simulink model "SensorFaultInj"  (R2014a)
settings: Solver=FixedStepDiscrete  SolverMode=SingleTasking  StartTime=0.0  StopTime=SimLength  FixedStep=SampleTime  RelTol=1e-3
values from neighbouring files (symbols this model uses):
  GlobalSeed = 10    [set_global_attr.m]
  SampleTime = 0.01    [set_global_attr.m]
  SimLength = 40    [set_global_attr.m]
undefined symbols (not defined in the file or in its folder): actMat, DiscIntNeverNeededParam
libraries: simulink x16, dspswit3 x10
(part 1 of 4)
settings Model: Creator=Maik  LastModifiedBy=Maik
settings DataIOCC: SaveOutput=off  SaveTime=off
settings DebuggingCC: UnconnectedOutputMsg=none  BusObjectLabelMismatch=none  StateNameClashWarn=warning

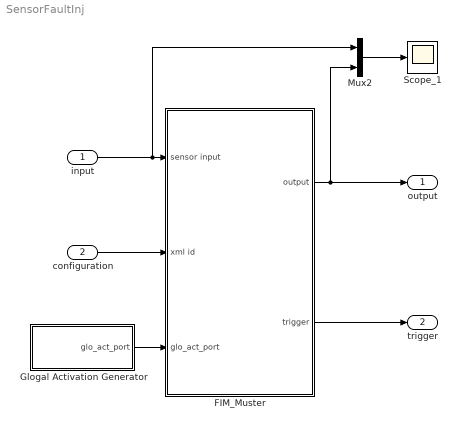
== system SensorFaultInj ==
  "input " : Inport  SampleTime=SampleTime
  configuration : Inport  Port=2  OutDataTypeStr=single  SampleTime=SampleTime
  FIM_Muster : Subsystem
  Glogal Activation Generator : Subsystem  TreatAsAtomicUnit=on
  Mux2 : Mux  Inputs=2
  Scope_1 : Scope
      settings: TimeRange=40  YMin=0.1  YMax=0.24  SaveName=SensordataEva01  MaxDataPoints=50000
  output : Outport
  trigger : Outport  Port=2  OutDataTypeStr=Bus: TriggerBus  SampleTime=SampleTime
  wires:
  Mux2/1 -> Scope_1/1
  FIM_Muster/1(output) -> Mux2/2, output/1
  "input "/1 -> Mux2/1, FIM_Muster/1(sensor input)
  configuration/1 -> FIM_Muster/2(xml id)
  Glogal Activation Generator/1(glo_act_port) -> FIM_Muster/3(glo_act_port)
  FIM_Muster/2(trigger) -> trigger/1

== system SensorFaultInj/FIM_Muster ==
  sensor input : Inport
  xml id : Inport  Port=2  SampleTime=SampleTime
  glo_act_port : Inport  Port=3
  Fault Injection Modul : Subsystem
  Local Activation Generator : Subsystem
  Parser Modul : Subsystem
  logger : Subsystem
  trigger signal generation : Subsystem
  output : Outport
  trigger : Outport  Port=2
  wires:
  Parser Modul/1(schedule_port) -> Local Activation Generator/1(schedule_port), trigger signal generation/1(schedule), Fault Injection Modul/2(schedule_port)
  Parser Modul/2(occurrnce_port) -> Local Activation Generator/2(occurrence_port)
  Local Activation Generator/1(activation_port) -> Parser Modul/2("actiavtion_vector "), trigger signal generation/2(activation), Fault Injection Modul/3(activation_port)
  Fault Injection Modul/1(Out1) -> logger/2("input "), output/1
  sensor input/1 -> Fault Injection Modul/1(sensor input)
  xml id/1 -> logger/1(xml_id), Parser Modul/1(xml id)
  Parser Modul/3(parameter_port) -> Local Activation Generator/3("param_port "), Fault Injection Modul/4(parameter_port)
  Fault Injection Modul/2("amplitude_port ") -> logger/4("amp_port ")
  Local Activation Generator/2(log_port) -> logger/3("act_port ")
  glo_act_port/1 -> Local Activation Generator/4(glo_act_port)
  trigger signal generation/1(Out1) -> trigger/1

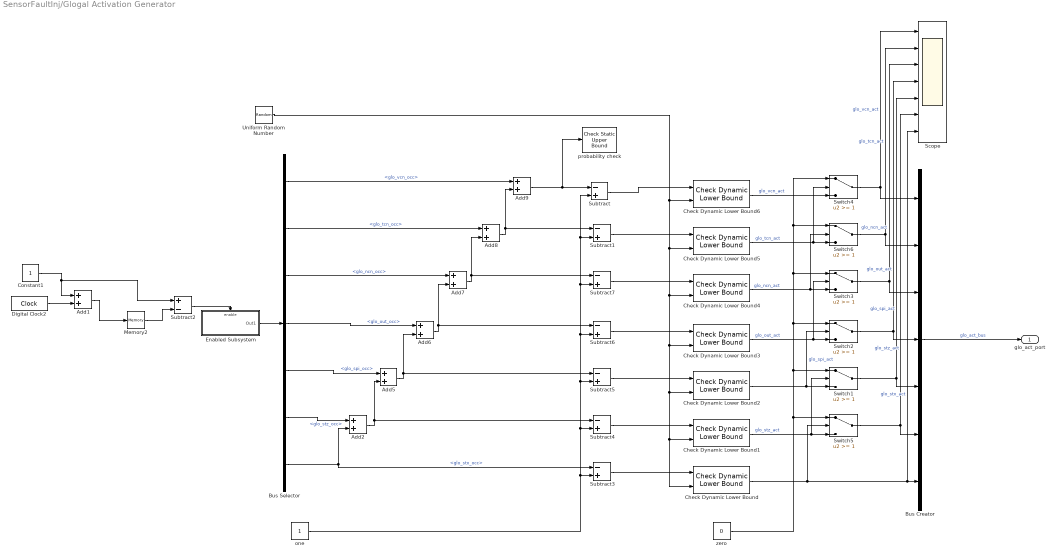
== system SensorFaultInj/Glogal Activation Generator ==
  Add{1..2,5..9} (7 alike) : Sum
  Bus Creator : BusCreator  Inputs=7
  Bus Selector : BusSelector  OutputSignals=glo_vcn_occ,glo_tcn_occ,glo_ncn_occ,glo_out_occ,glo_spi_occ,glo_stz_occ,glo_stx_occ
  Check Dynamic Lower Bound{,1..6} (7 alike) : simulink/Model Verification/Check Dynamic  Lower Bound  Description=min < sig  Enabled=off  stopWhenAssertionFail=off  export=on  icon=graphic
  Constant1 : Constant
  Digital Clock2 : DigitalClock  SampleTime=SampleTime
  Enabled Subsystem : Subsystem  TreatAsAtomicUnit=on
  Memory2 : Memory
  Scope : Scope  NumInputPorts=7
      settings: YMin=-5~-5~-5~-5~-5~-5~-5  YMax=5~5~5~5~5~5~5  SaveName=ScopeData10
  Subtract{,1,3..7} (7 alike) : Sum  Inputs=-+
  Subtract2 : Sum  Inputs=+-
  Switch{1..6} (6 alike) : Switch  Threshold=1
      settings: LockScale=on
  Uniform Random Number : UniformRandomNumber  Seed=GlobalSeed  SampleTime=SampleTime
  one : Constant
  probability check : simulink/Model Verification/Check Static  Upper Bound  Description=u <= 1  max=1  max_included=on  enabled=on  stopWhenAssertionFail=on  export=off  icon=graphic
  zero : Constant  Value=0
  glo_act_port : Outport
  wires:
  Bus Selector/7 -> Subtract3/1, Add2/2  "<glo_stx_occ>"
  Bus Selector/6 -> Add2/1  "<glo_stz_occ>"
  Add5/1 -> Add6/2, Subtract5/1
  Bus Selector/5 -> Add5/1  "<glo_spi_occ>"
  Bus Selector/4 -> Add6/1  "<glo_out_occ>"
  Add6/1 -> Add7/2, Subtract6/1
  Add7/1 -> Add8/2, Subtract7/1
  Bus Selector/3 -> Add7/1  "<glo_ncn_occ>"
  Bus Selector/2 -> Add8/1  "<glo_tcn_occ>"
  Add8/1 -> Add9/2, Subtract1/1
  Bus Selector/1 -> Add9/1  "<glo_vcn_occ>"
  Uniform Random Number/1 -> Check Dynamic Lower Bound/2, Check Dynamic Lower Bound1/2, Check Dynamic Lower Bound2/2, Check Dynamic Lower Bound3/2, Check Dynamic Lower Bound4/2, Check Dynamic Lower Bound5/2, Check Dynamic Lower Bound6/2
  Subtract/1 -> Check Dynamic Lower Bound6/1
  Add9/1 -> probability check/1, Subtract/1
  Subtract1/1 -> Check Dynamic Lower Bound5/1
  Subtract7/1 -> Check Dynamic Lower Bound4/1
  Subtract6/1 -> Check Dynamic Lower Bound3/1
  Subtract5/1 -> Check Dynamic Lower Bound2/1
  Subtract4/1 -> Check Dynamic Lower Bound1/1
  Subtract3/1 -> Check Dynamic Lower Bound/1
  one/1 -> Subtract/2, Subtract1/2, Subtract7/2, Subtract6/2, Subtract5/2, Subtract4/2, Subtract3/2
  Add2/1 -> Subtract4/1, Add5/2
  Check Dynamic Lower Bound/1 -> Switch5/2, Scope/7, Bus Creator/7  "glo_stx_act"
  Switch5/1 -> Bus Creator/6, Scope/6  "glo_stz_act"
  Switch1/1 -> Bus Creator/5, Scope/5  "glo_spi_act"
  Switch2/1 -> Bus Creator/4, Scope/4  "glo_out_act"
  Switch3/1 -> Bus Creator/3, Scope/3  "glo_ncn_act"
  Switch6/1 -> Bus Creator/2, Scope/2  "glo_tcn_act"
  Switch4/1 -> Bus Creator/1, Scope/1  "glo_vcn_act"
  Bus Creator/1 -> glo_act_port/1  "glo_act_bus"
  Check Dynamic Lower Bound1/1 -> Switch1/2, Switch5/3  "glo_stz_act"
  zero/1 -> Switch3/1, Switch6/1, Switch4/1, Switch2/1, Switch1/1, Switch5/1
  Check Dynamic Lower Bound2/1 -> Switch2/2, Switch1/3  "glo_spi_act"
  Check Dynamic Lower Bound3/1 -> Switch3/2, Switch2/3  "glo_out_act"
  Check Dynamic Lower Bound4/1 -> Switch6/2, Switch3/3  "glo_ncn_act"
  Check Dynamic Lower Bound5/1 -> Switch4/2, Switch6/3  "glo_tcn_act"
  Check Dynamic Lower Bound6/1 -> Switch4/3  "glo_vcn_act"
  Digital Clock2/1 -> Add1/2
  Memory2/1 -> Subtract2/2
  Constant1/1 -> Add1/1, Subtract2/1
  Add1/1 -> Memory2/1
  Subtract2/1 -> Enabled Subsystem/Enable
  Enabled Subsystem/1(Out1) -> Bus Selector/1

== system SensorFaultInj/FIM_Muster/Fault Injection Modul ==
  sensor input : Inport
  schedule_port : Inport  Port=2
  activation_port : Inport  Port=3
  parameter_port : Inport  Port=4
  AFI - additive faults injection : Subsystem
  Bus Creator : BusCreator  Inputs=3
  FFI - functional fault injection : Subsystem
  MFI - multiplicative fault injection : Subsystem
  activation bus creator : Subsystem
  schedule bus creator : Subsystem
  schedule bus creator1 : Subsystem
  Out1 : Outport
  "amplitude_port " : Outport  Port=2
  wires:
  MFI - multiplicative fault injection/1(output) -> AFI - additive faults injection/1(input)
  FFI - functional fault injection/1(output) -> Out1/1
  AFI - additive faults injection/1(output) -> FFI - functional fault injection/1(input)
  sensor input/1 -> MFI - multiplicative fault injection/1(In1)
  activation_port/1 -> activation bus creator/1(act_port)
  schedule_port/1 -> schedule bus creator/1(schedule_port)
  schedule bus creator/1(mfi_sched_port) -> MFI - multiplicative fault injection/2(sched_port)
  activation bus creator/1(mfi_act_port) -> MFI - multiplicative fault injection/3(act_port)
  schedule bus creator1/1(mfi_sched_port) -> MFI - multiplicative fault injection/4(param_port)
  schedule bus creator/2(afi_sched_port) -> AFI - additive faults injection/2(sched_bus)
  activation bus creator/2(afi_act_port) -> AFI - additive faults injection/3(act_bus)
  schedule bus creator1/2(afi_sched_port) -> AFI - additive faults injection/4(param_bus)
  schedule bus creator/3(ffi_sched_port) -> FFI - functional fault injection/2(schedule_port)
  schedule bus creator1/3(ffi_sched_port) -> FFI - functional fault injection/3(param_port)
  parameter_port/1 -> schedule bus creator1/1(schedule_port)
  MFI - multiplicative fault injection/2("amplitude_port ") -> Bus Creator/1
  AFI - additive faults injection/2("amplitude_bus ") -> Bus Creator/2
  Bus Creator/1 -> "amplitude_port "/1  "ampl_bus"
  FFI - functional fault injection/2(amplitude_port) -> Bus Creator/3

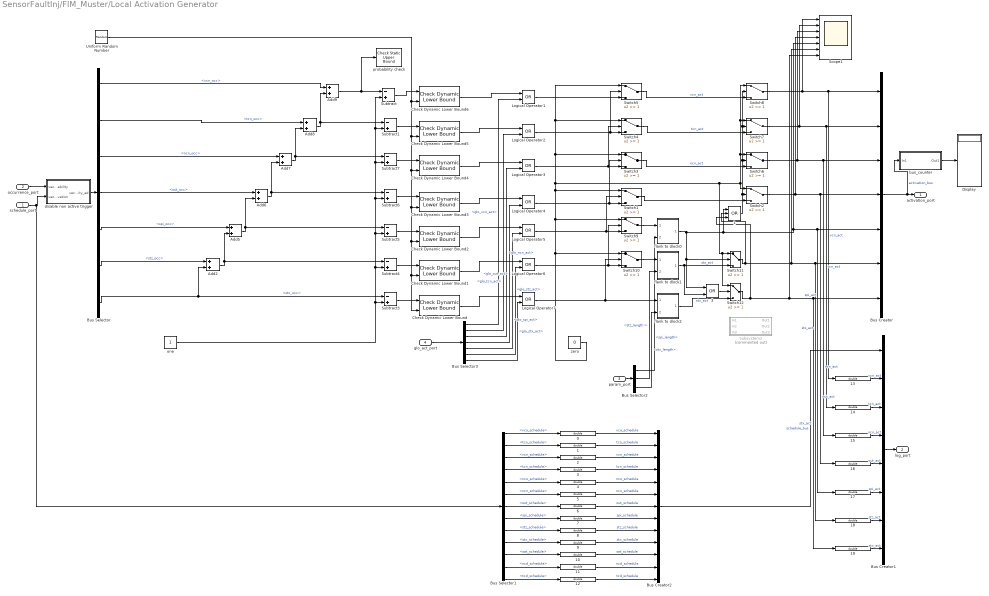
== system SensorFaultInj/FIM_Muster/Local Activation Generator ==
  schedule_port : Inport
  occurrence_port : Inport  Port=2
  "param_port " : Inport  Port=3
  glo_act_port : Inport  Port=4
  " 1" : Logic  Operator=OR  Inputs=3  AllPortsSameDT=off  OutDataTypeStr=boolean
  " 3" : Logic  Operator=OR  AllPortsSameDT=off  OutDataTypeStr=boolean
  {0..19} (20 alike) : DataTypeConversion  OutDataTypeStr=double
  Add{2,5..9} (6 alike) : Sum
  Bus Creator : BusCreator  Inputs=7
  Bus Creator1 : BusCreator  Inputs=8
  Bus Creator2 : BusCreator  Inputs=13
  Bus Selector : BusSelector  OutputSignals=vcn_occ,tcn_occ,ncn_occ,out_occ,spi_occ,stz_occ,stx_occ
  Bus Selector1 : BusSelector  OutputSignals=vco_schedule,tco_schedule,vcn_schedule,tcn_schedule,nco_schedule,ncn_schedule,out_schedule,spi_schedule,stz_schedule,stx_schedule,sat_schedule,ncd_schedule,tcd_schedule
  Bus Selector2 : BusSelector  OutputSignals=parameter_bus.spi_param_bus.spi_length,parameter_bus.stz_length ,parameter_bus.stx_param_bus.stx_length
  Bus Selector3 : BusSelector  OutputSignals=glo_vcn_act,glo_tcn_act,glo_ncn_act,glo_out_act,glo_spi_act,glo_stz_act,glo_stx_act
  Check Dynamic Lower Bound{,1..6} (7 alike) : simulink/Model Verification/Check Dynamic  Lower Bound  Description=min < sig  Enabled=off  stopWhenAssertionFail=off  export=on  icon=graphic
  Display : Display
  Logical Operator{1..7} (7 alike) : Logic  Operator=OR  AllPortsSameDT=off  OutDataTypeStr=boolean
  Scope1 : Scope  NumInputPorts=7
      settings: TimeRange=1  YMin=-1~0~-5~-5~-5~-5~-5  YMax=1~1~5~5~5~5~5  SaveName=ScopeData23  MaxDataPoints=50000
  Subsystem2 : Subsystem  Commented=on
  Subtract{,1,3..7} (7 alike) : Sum  Inputs=-+
  Switch{1..12} (12 alike) : Switch  Threshold=1
      Switch1 settings: LockScale=on
      Switch10 settings: LockScale=on
      Switch5 settings: LockScale=on
      Switch9 settings: LockScale=on
  Uniform Random Number : UniformRandomNumber  Minimum=0  Seed=1  SampleTime=SampleTime
  bus_counter : Subsystem
  disable non active trigger : Subsystem
  flank to dlock0 : Subsystem
  flank to dlock1 : Subsystem
  flank to dlock2 : Subsystem
  one : Constant
  probability check : simulink/Model Verification/Check Static  Upper Bound  Description=u <= 1  max=1  max_included=on  enabled=on  stopWhenAssertionFail=on  export=off  icon=graphic
  zero : Constant  Value=0  OutDataTypeStr=boolean
  activation_port : Outport
  log_port : Outport  Port=2
  wires:
  Bus Selector/7 -> Add2/2, Subtract3/1  "<stx_occ>"
  Bus Selector/6 -> Add2/1  "<stz_occ>"
  Add5/1 -> Add6/2, Subtract5/1
  Bus Selector/5 -> Add5/1  "<spi_occ>"
  Bus Selector/4 -> Add6/1  "<out_occ>"
  Add6/1 -> Add7/2, Subtract6/1
  Add7/1 -> Add8/2, Subtract7/1
  Bus Selector/3 -> Add7/1  "<ncn_occ>"
  Bus Selector/2 -> Add8/1  "<tcn_occ>"
  Add8/1 -> Add9/2, Subtract1/1
  Bus Selector/1 -> Add9/1  "<vcn_occ>"
  Subtract/1 -> Check Dynamic Lower Bound6/1
  Add9/1 -> probability check/1, Subtract/1
  Subtract1/1 -> Check Dynamic Lower Bound5/1
  Subtract7/1 -> Check Dynamic Lower Bound4/1
  Subtract6/1 -> Check Dynamic Lower Bound3/1
  Subtract5/1 -> Check Dynamic Lower Bound2/1
  Subtract4/1 -> Check Dynamic Lower Bound1/1
  Subtract3/1 -> Check Dynamic Lower Bound/1
  one/1 -> Subtract/2, Subtract1/2, Subtract7/2, Subtract6/2, Subtract5/2, Subtract4/2, Subtract3/2
  zero/1 -> Switch1/1, Switch12/1, Switch11/1, Switch2/1, Switch8/1, Switch7/1, Switch6/1, Switch3/1, Switch4/1, Switch5/1, Switch9/1, Switch10/1
  Switch8/1 -> Scope1/1, 13/1, Bus Creator/1  "vcn_act"
  Switch7/1 -> Scope1/2, 14/1, Bus Creator/2  "tcn_act"
  Switch6/1 -> Scope1/3, 15/1, Bus Creator/3  "ncn_act"
  Switch2/1 -> 16/1, Bus Creator/4, Scope1/4  "out_act"
  flank to dlock0/1(block) -> " 1"/1, Scope1/5, 17/1, Bus Creator/5, Switch11/2, " 3"/1  "spi_act"
  Switch11/1 -> " 1"/2, Scope1/6, 18/1, Bus Creator/6  "stz_act"
  Bus Creator/1 -> activation_port/1, bus_counter/1(In1)  "activation_bus"
  occurrence_port/1 -> disable non active trigger/1(vec_probability)
  schedule_port/1 -> Bus Selector1/1, disable non active trigger/2(vec_activation)
  Add2/1 -> Subtract4/1, Add5/2
  Switch12/1 -> " 1"/3, Scope1/7, 19/1, Bus Creator/7  "stx_act"
  disable non active trigger/1(vec_probability_ad) -> Bus Selector/1
  Bus Creator1/1 -> log_port/1
  Bus Selector1/1 -> 0/1  "<vco_schedule>"
  3/1 -> Bus Creator2/4  "tcn_schedule"
  0/1 -> Bus Creator2/1  "vco_schedule"
  4/1 -> Bus Creator2/5  "nco_schedule"
  1/1 -> Bus Creator2/2  "tco_schedule"
  2/1 -> Bus Creator2/3  "vcn_schedule"
  5/1 -> Bus Creator2/6  "ncn_schedule"
  6/1 -> Bus Creator2/7  "out_schedule"
  12/1 -> Bus Creator2/13  "tcd_schedule"
  7/1 -> Bus Creator2/8  "spi_schedule"
  8/1 -> Bus Creator2/9  "stz_schedule"
  9/1 -> Bus Creator2/10  "stx_schedule"
  10/1 -> Bus Creator2/11  "sat_schedule"
  11/1 -> Bus Creator2/12  "ncd_schedule"
  Bus Selector1/2 -> 1/1  "<tco_schedule>"
  Bus Selector1/3 -> 2/1  "<vcn_schedule>"
  Bus Selector1/4 -> 3/1  "<tcn_schedule>"
  Bus Selector1/5 -> 4/1  "<nco_schedule>"
  Bus Selector1/6 -> 5/1  "<ncn_schedule>"
  Bus Selector1/7 -> 6/1  "<out_schedule>"
  Bus Selector1/8 -> 7/1  "<spi_schedule>"
  Bus Selector1/9 -> 8/1  "<stz_schedule>"
  Bus Selector1/10 -> 9/1  "<stx_schedule>"
  Bus Selector1/11 -> 10/1  "<sat_schedule>"
  Bus Selector1/12 -> 11/1  "<ncd_schedule>"
  Bus Selector1/13 -> 12/1  "<tcd_schedule>"
  Bus Creator2/1 -> Bus Creator1/1  "schedule_bus"
  13/1 -> Bus Creator1/2  "vcn_act"
  14/1 -> Bus Creator1/3  "tcn_act"
  15/1 -> Bus Creator1/4  "ncn_act"
  16/1 -> Bus Creator1/5  "out_act"
  17/1 -> Bus Creator1/6  "spi_act"
  18/1 -> Bus Creator1/7  "stz_act"
  19/1 -> Bus Creator1/8  "stx_act"
  "param_port "/1 -> Bus Selector2/1
  Bus Selector2/1 -> flank to dlock0/2(delay)  "<spi_length>"
  Bus Selector2/2 -> flank to dlock1/2(delay)  "<stz_length >"
  Bus Selector2/3 -> flank to dlock2/2(delay)  "<stx_length>"
  Logical Operator1/1 -> Switch5/3
  Check Dynamic Lower Bound6/1 -> Logical Operator1/1
  Logical Operator3/1 -> Switch3/3, Switch4/2
  Logical Operator2/1 -> Switch5/2, Switch4/3
  Check Dynamic Lower Bound5/1 -> Logical Operator2/1
  Check Dynamic Lower Bound4/1 -> Logical Operator3/1
  Check Dynamic Lower Bound3/1 -> Logical Operator4/1
  Check Dynamic Lower Bound2/1 -> Logical Operator5/1
  Check Dynamic Lower Bound1/1 -> Logical Operator6/1
  Check Dynamic Lower Bound/1 -> Logical Operator7/1
  glo_act_port/1 -> Bus Selector3/1
  Bus Selector3/7 -> Logical Operator7/2  "<glo_stx_act>"
  Bus Selector3/6 -> Logical Operator6/2  "<glo_stz_act>"
  Bus Selector3/5 -> Logical Operator5/2  "<glo_spi_act>"
  Bus Selector3/4 -> Logical Operator4/2  "<glo_out_act>"
  Bus Selector3/3 -> Logical Operator3/2  "<glo_ncn_act>"
  Bus Selector3/2 -> Logical Operator2/2  "<glo_tcn_act>"
  Bus Selector3/1 -> Logical Operator1/2  "<glo_vcn_act>"
  bus_counter/1(Out1) -> Display/1
  Uniform Random Number/1 -> Check Dynamic Lower Bound4/2, Check Dynamic Lower Bound3/2, Check Dynamic Lower Bound2/2, Check Dynamic Lower Bound1/2, Check Dynamic Lower Bound/2, Check Dynamic Lower Bound5/2, Check Dynamic Lower Bound6/2
  " 1"/1 -> Switch6/2, Switch8/2, Switch7/2, Switch2/2
  Switch3/1 -> Switch6/3  "ncn_act"
  Switch4/1 -> Switch7/3  "tcn_act"
  Switch5/1 -> Switch8/3  "vcn_act"
  Switch1/1 -> Switch2/3
  Logical Operator4/1 -> Switch3/2, Switch1/3
  Logical Operator5/1 -> Switch1/2, Switch9/3
  Logical Operator6/1 -> Switch9/2, Switch10/3
  Logical Operator7/1 -> flank to dlock2/1(flank), Switch10/2
  Switch10/1 -> flank to dlock1/1(flank)
  Switch9/1 -> flank to dlock0/1(flank)
  flank to dlock2/1(block) -> Switch12/3  "stx_act"
  flank to dlock1/1(block) -> " 3"/2, Switch11/3  "stz_act"
  " 3"/1 -> Switch12/2

== system SensorFaultInj/FIM_Muster/Parser Modul ==
  xml id : Inport
  "actiavtion_vector " : Inport  Port=2
  Bus Creator : BusCreator  Inputs=2
  Fault Parameter Parser : Subsystem
  "Occurence Parser " : Subsystem  Commented=on
  "Schedule Parser and Generator " : Subsystem
  "actication matrix parser " : Subsystem
  activation_vec : Display
  parameter_vec : Display
  schedule : Scope
      settings: SaveName=ScopeData2
  schedule_port : Outport
  occurrnce_port : Outport  Port=2
  parameter_port : Outport  Port=3
  wires:
  "Schedule Parser and Generator "/1(Out1) -> schedule/1, activation_vec/1, schedule_port/1
  xml id/1 -> "Schedule Parser and Generator "/1(In1), Fault Parameter Parser/1(In1), Bus Creator/2, "Occurence Parser "/1(In1)  "xml_id"
  Fault Parameter Parser/1(Out1) -> parameter_vec/1, Bus Creator/1  "parameter_bus"
  Bus Creator/1 -> parameter_port/1
  "actiavtion_vector "/1 -> "actication matrix parser "/1(In1)
  "actication matrix parser "/1(Out1) -> occurrnce_port/1

== system SensorFaultInj/FIM_Muster/logger ==
  xml_id : Inport
  "input " : Inport  Port=2
  "act_port " : Inport  Port=3
  "amp_port " : Inport  Port=4
  Bus Creator : BusCreator  Inputs=13
  Bus Creator1 : BusCreator  Inputs=13
  Bus Selector : BusSelector  OutputSignals=schedule_bus.vco_schedule,schedule_bus.tco_schedule,vcn_act,tcn_act,schedule_bus.nco_schedule,ncn_act,out_act,spi_act,stz_act,stx_act,schedule_bus.sat_schedule,schedule_bus.ncd_schedule,schedule_bus.tcd_schedule
  Bus Selector1 : BusSelector  OutputSignals=mfi_amp_bus.vco_ampl,mfi_amp_bus.tco_ampl,mfi_amp_bus.vcn_ampl,mfi_amp_bus.tcn_ampl,afi_ampl_bus.nco_ampl,afi_ampl_bus.ncn_ampl,afi_ampl_bus.out_ampl,afi_ampl_bus.spike_ampl,afi_ampl_bus.stz_ampl,afi_ampl_bus.stx_ampl,ffi_ampl_bus.sat_ampl,ffi_ampl_bus.ncd_ampl,ffi_ampl_bus.tcd_ampl
  Constant1 : Constant
  Discrete-Time Integrator : DiscreteIntegrator  SampleTime=SampleTime  ICPrevOutput=DiscIntNeverNeededParam  ICPrevScaledInput=DiscIntNeverNeededParam
  Display : Display
  Display1 : Display
  ex_sfun_logger : S-Function  FunctionName=ex_sfun_logger  EnableBusSupport=off  mask(Legacy Function){SFunctionSpec=single y1 = logger(single u1, double u2, double u3, double u4[], double u5[]), ShowSpec=on}
      mask prompts: ShowSpec "Display function specification"
      mask help:
      | This block allows you to call the legacy functions specified by the following Legacy Code Tool definition:
      | def.SFunctionName = 'ex_sfun_logger';
      | def.OutputFcnSpec = 'single y1 = logger(single u1, double u2, double u3, double u4[], double u5[])';
      | def.HeaderFiles = {'logger.hpp'};
      | def.SourceFiles = {'logger.cpp'};
      | def.Options.language = 'C++';
      mask Help: <p>This block was generated automatically by the Legacy Code Tool. For detailed help on this tool, call<a href="matlab:legacy_code('help')"> legacy_code('help')</a>.</p>
      mask Callback ShowSpec:
      | if strcmp(get_param(gcbh, 'ShowSpec'), 'on')
      |   set_param(gcbh, 'MaskDisplay', sprintf('fprintf(''%s'');', get_param(gcbh, 'SFunctionSpec')));
      | else
      |   set_param(gcbh, 'MaskDisplay', sprintf('fprintf(''%s'');', get_param(gcbh, 'FunctionName')));
      | end
      mask Display: fprintf('single y1 = logger(single u1, double u2, double u3, double u4[], double u5[])');
  wires:
  "act_port "/1 -> Bus Selector/1
  "amp_port "/1 -> Bus Selector1/1
  Bus Selector1/2 -> Bus Creator1/2  "<tco_ampl>"
  Bus Selector1/3 -> Bus Creator1/3  "<vcn_ampl>"
  Bus Selector1/4 -> Bus Creator1/4  "<tcn_ampl>"
  Bus Selector1/6 -> Bus Creator1/6  "<ncn_ampl>"
  Bus Selector1/7 -> Bus Creator1/7  "<out_ampl>"
  Bus Selector1/8 -> Bus Creator1/8  "<spike_ampl>"
  Bus Selector1/1 -> Bus Creator1/1  "<vco_ampl>"
  Bus Selector1/5 -> Bus Creator1/5  "<nco_ampl>"
  Bus Selector1/9 -> Bus Creator1/9  "<stz_ampl>"
  Bus Selector1/10 -> Bus Creator1/10  "<stx_ampl>"
  Bus Selector1/13 -> Bus Creator1/13  "<tcd_ampl>"
  Bus Selector1/12 -> Bus Creator1/12  "<ncd_ampl>"
  Bus Selector1/11 -> Bus Creator1/11  "<sat_ampl>"
  Bus Creator/1 -> Display/1, ex_sfun_logger/4
  Bus Creator1/1 -> ex_sfun_logger/5, Display1/1
  xml_id/1 -> ex_sfun_logger/1
  Constant1/1 -> Discrete-Time Integrator/1
  Bus Selector/11 -> Bus Creator/11  "<sat_schedule>"
  Bus Selector/12 -> Bus Creator/12  "<ncd_schedule>"
  Bus Selector/13 -> Bus Creator/13  "<tcd_schedule>"
  Bus Selector/3 -> Bus Creator/3  "<vcn_act>"
  Bus Selector/4 -> Bus Creator/4  "<tcn_act>"
  Bus Selector/5 -> Bus Creator/5  "<nco_schedule>"
  Bus Selector/6 -> Bus Creator/6  "<ncn_act>"
  Bus Selector/8 -> Bus Creator/8  "<spi_act>"
  Bus Selector/10 -> Bus Creator/10  "<stx_act>"
  Bus Selector/9 -> Bus Creator/9  "<stz_act>"
  Bus Selector/7 -> Bus Creator/7  "<out_act>"
  Bus Selector/1 -> Bus Creator/1  "<vco_schedule>"
  Bus Selector/2 -> Bus Creator/2  "<tco_schedule>"
  "input "/1 -> ex_sfun_logger/3
  Discrete-Time Integrator/1 -> ex_sfun_logger/2

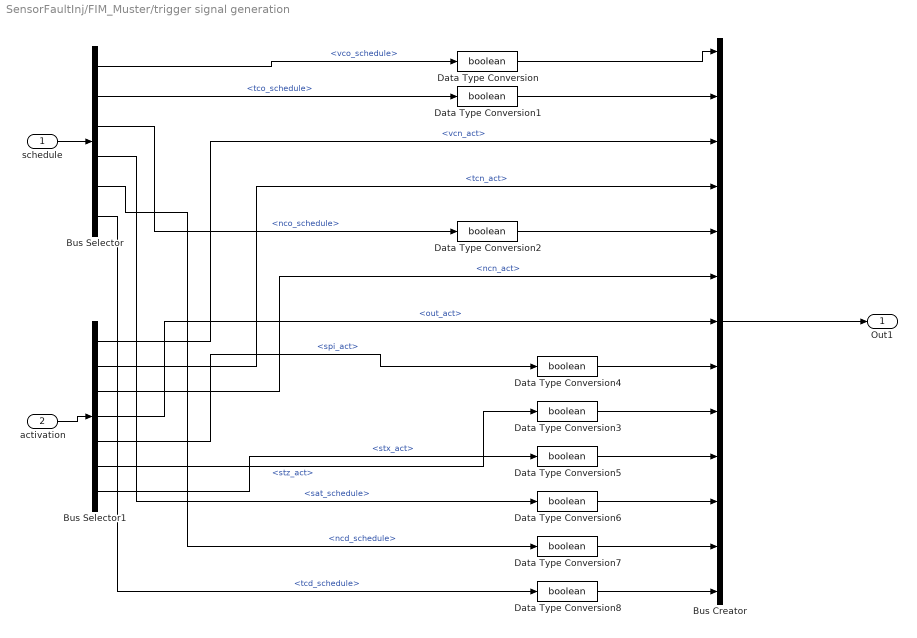
== system SensorFaultInj/FIM_Muster/trigger signal generation ==
  schedule : Inport
  activation : Inport  Port=2
  Bus Creator : BusCreator  Inputs=13
  Bus Selector : BusSelector  OutputSignals=vco_schedule,tco_schedule,nco_schedule,sat_schedule,ncd_schedule,tcd_schedule
  Bus Selector1 : BusSelector  OutputSignals=vcn_act,tcn_act,ncn_act,out_act,spi_act,stz_act,stx_act
  Data Type Conversion{,1..8} (9 alike) : DataTypeConversion  OutDataTypeStr=boolean
  Out1 : Outport
  wires:
  schedule/1 -> Bus Selector/1
  activation/1 -> Bus Selector1/1
  Bus Selector/1 -> Data Type Conversion/1  "<vco_schedule>"
  Bus Selector/2 -> Data Type Conversion1/1  "<tco_schedule>"
  Bus Selector1/1 -> Bus Creator/3  "<vcn_act>"
  Bus Selector1/2 -> Bus Creator/4  "<tcn_act>"
  Bus Selector/3 -> Data Type Conversion2/1  "<nco_schedule>"
  Bus Selector1/3 -> Bus Creator/6  "<ncn_act>"
  Bus Selector1/4 -> Bus Creator/7  "<out_act>"
  Bus Selector1/5 -> Data Type Conversion4/1  "<spi_act>"
  Bus Selector1/6 -> Data Type Conversion3/1  "<stz_act>"
  Bus Selector1/7 -> Data Type Conversion5/1  "<stx_act>"
  Bus Selector/4 -> Data Type Conversion6/1  "<sat_schedule>"
  Bus Selector/5 -> Data Type Conversion7/1  "<ncd_schedule>"
  Bus Selector/6 -> Data Type Conversion8/1  "<tcd_schedule>"
  Bus Creator/1 -> Out1/1
  Data Type Conversion/1 -> Bus Creator/1
  Data Type Conversion1/1 -> Bus Creator/2
  Data Type Conversion2/1 -> Bus Creator/5
  Data Type Conversion3/1 -> Bus Creator/9
  Data Type Conversion4/1 -> Bus Creator/8
  Data Type Conversion5/1 -> Bus Creator/10
  Data Type Conversion6/1 -> Bus Creator/11
  Data Type Conversion7/1 -> Bus Creator/12
  Data Type Conversion8/1 -> Bus Creator/13

== system SensorFaultInj/Glogal Activation Generator/Enabled Subsystem ==
  Enable : EnablePort
  Bus Creator : BusCreator  Inputs=7
  global parser2 : Subsystem
  global parser3 : Subsystem
  global parser5 : Subsystem
  global parser6 : Subsystem
  global parser7 : Subsystem
  global parser8 : Subsystem
  global parser9 : Subsystem
  Out1 : Outport
  wires:
  Bus Creator/1 -> Out1/1  "occurrence_bus"
  global parser3/1(occ) -> Bus Creator/2
  global parser8/1(occ) -> Bus Creator/6
  global parser7/1(occ) -> Bus Creator/5
  global parser2/1(occ) -> Bus Creator/1
  global parser5/1(occ) -> Bus Creator/3
  global parser9/1(occ) -> Bus Creator/7
  global parser6/1(occ) -> Bus Creator/4

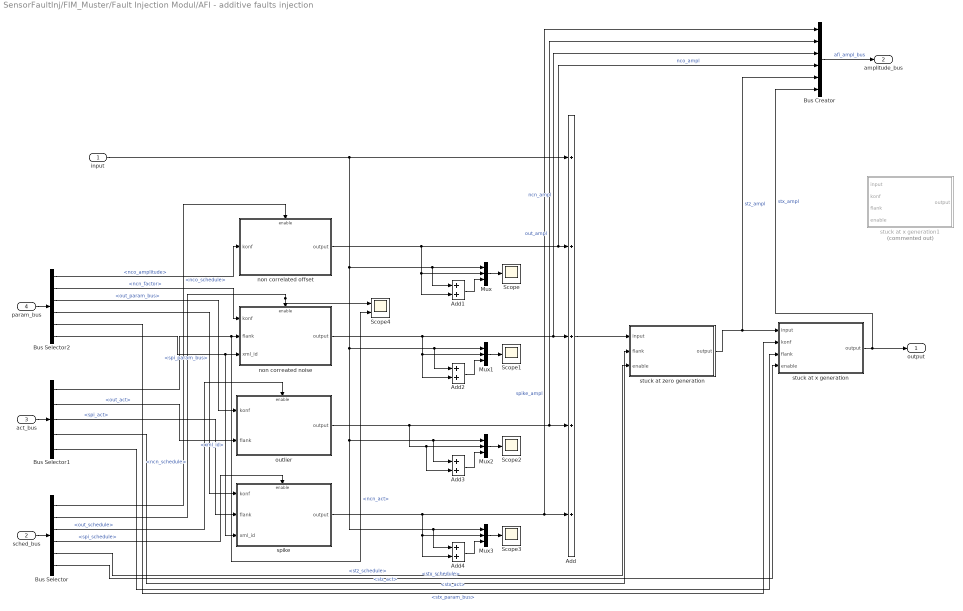
== system SensorFaultInj/FIM_Muster/Fault Injection Modul/AFI - additive faults injection ==
  input : Inport
  sched_bus : Inport  Port=2
  act_bus : Inport  Port=3
  param_bus : Inport  Port=4
  Add : Sum  Inputs=+++++
  Add{1..4} (4 alike) : Sum
  Bus Creator : BusCreator  Inputs=6
  Bus Selector : BusSelector  OutputSignals=nco_schedule,ncn_schedule,out_schedule,spi_schedule,stz_schedule,stx_schedule
  Bus Selector1 : BusSelector  OutputSignals=ncn_act,out_act,spi_act,stz_act,stx_act
  Bus Selector2 : BusSelector  OutputSignals=nco_amplitude,ncn_factor,out_param_bus,spi_param_bus,stx_param_bus,xml_id
  Mux{,1..3} (4 alike) : Mux  Inputs=3
  Scope{,1..3} (4 alike) : Scope
      Scope settings: YMin=-70  YMax=70  SaveName=ScopeData14  MaxDataPoints=10000
      Scope1 settings: YMin=-50  YMax=55  SaveName=ScopeData15
      Scope2 settings: YMin=-70  YMax=70  SaveName=ScopeData16
      Scope3 settings: YMin=-50  YMax=60  SaveName=ScopeData17
  Scope4 : Scope  NumInputPorts=2
      settings: YMin=-70~-5  YMax=70~5  SaveName=ScopeData28
  non correated noise : Subsystem
  non correlated offset : Subsystem
  outlier : Subsystem
  spike : Subsystem
  stuck at x generation : Subsystem
  stuck at x generation1 : Subsystem  Commented=on
  stuck at zero generation : Subsystem
  output : Outport
  "amplitude_bus " : Outport  Port=2
  wires:
  input/1 -> Add1/1, Mux/1, Add4/1, Mux3/1, Add3/1, Mux2/1, Add2/1, Mux1/1, Add/1
  non correlated offset/1(output) -> Add1/2, Mux/2, Bus Creator/4, Add/2  "nco_ampl"
  non correated noise/1(output) -> Add2/2, Mux1/2, Bus Creator/3, Add/3  "ncn_ampl"
  outlier/1(output) -> Add3/2, Mux2/2, Bus Creator/2, Add/4  "out_ampl"
  spike/1(output) -> Bus Creator/1, Add/5, Add4/2, Mux3/2  "spike_ampl"
  Mux/1 -> Scope/1
  Mux1/1 -> Scope1/1
  Mux2/1 -> Scope2/1
  Mux3/1 -> Scope3/1
  Add1/1 -> Mux/3
  Add2/1 -> Mux1/3
  Add3/1 -> Mux2/3
  Add4/1 -> Mux3/3
  Add/1 -> stuck at zero generation/1(input)
  stuck at x generation/1(output) -> Bus Creator/6, output/1  "stx_ampl"
  stuck at zero generation/1(output) -> Bus Creator/5, stuck at x generation/1(input)  "stz_ampl"
  sched_bus/1 -> Bus Selector/1
  Bus Selector/1 -> non correlated offset/Enable  "<nco_schedule>"
  Bus Selector/2 -> Scope4/1, non correated noise/Enable  "<ncn_schedule>"
  Bus Selector/5 -> stuck at zero generation/3(enable)  "<stz_schedule>"
  Bus Selector/6 -> stuck at x generation/4(enable)  "<stx_schedule>"
  act_bus/1 -> Bus Selector1/1
  Bus Selector1/1 -> Scope4/2, non correated noise/2(flank)  "<ncn_act>"
  Bus Selector1/2 -> outlier/2(flank)  "<out_act>"
  Bus Selector1/3 -> spike/2(flank)  "<spi_act>"
  Bus Selector1/4 -> stuck at zero generation/2(flank)  "<stz_act>"
  Bus Selector1/5 -> stuck at x generation/3(flank)  "<stx_act>"
  param_bus/1 -> Bus Selector2/1
  Bus Selector2/1 -> non correlated offset/1(konf)  "<nco_amplitude>"
  Bus Selector2/2 -> non correated noise/1("konf ")  "<ncn_factor>"
  Bus Selector2/3 -> outlier/1(konf)  "<out_param_bus>"
  Bus Selector2/4 -> spike/1(konf)  "<spi_param_bus>"
  Bus Selector2/5 -> stuck at x generation/2(konf)  "<stx_param_bus>"
  Bus Selector2/6 -> spike/3(xml_id), non correated noise/3(xml_id)  "<xml_id>"
  Bus Creator/1 -> "amplitude_bus "/1  "afi_ampl_bus"
  Bus Selector/3 -> outlier/Enable  "<out_schedule>"
  Bus Selector/4 -> spike/Enable  "<spi_schedule>"

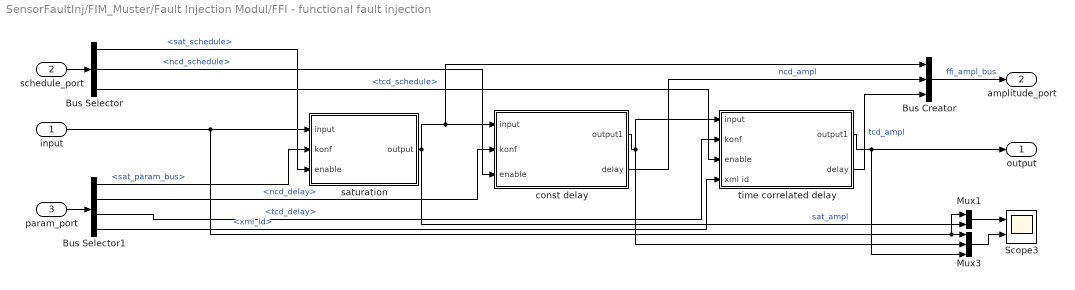
== system SensorFaultInj/FIM_Muster/Fault Injection Modul/FFI - functional fault injection ==
  input : Inport
  schedule_port : Inport  Port=2
  param_port : Inport  Port=3
  Bus Creator : BusCreator  Inputs=3
  Bus Selector : BusSelector  OutputSignals=sat_schedule,ncd_schedule,tcd_schedule
  Bus Selector1 : BusSelector  OutputSignals=sat_param_bus,ncd_delay,tcd_delay,xml_id
  Mux1 : Mux  Inputs=2
  Mux3 : Mux  Inputs=3
  Scope3 : Scope  NumInputPorts=2
      settings: YMin=-50~-50  YMax=50~50  SaveName=ScopeData6
  "const delay " : Subsystem
  saturation : Subsystem
  "time correlated delay " : Subsystem
  output : Outport
  amplitude_port : Outport  Port=2
  wires:
  input/1 -> Mux3/1, Mux1/1, saturation/1(input)
  Mux1/1 -> Scope3/1
  Mux3/1 -> Scope3/2
  saturation/1(output) -> Mux1/2, Bus Creator/1, "const delay "/1(input)  "sat_ampl"
  "const delay "/1(output1) -> "time correlated delay "/1(input), Mux3/2
  "time correlated delay "/1(output1) -> Mux3/3, output/1
  schedule_port/1 -> Bus Selector/1
  param_port/1 -> Bus Selector1/1
  Bus Selector1/4 -> "time correlated delay "/4(xml id)  "<xml_id>"
  Bus Selector1/3 -> "time correlated delay "/2(konf)  "<tcd_delay>"
  Bus Selector1/1 -> saturation/2("konf ")  "<sat_param_bus>"
  Bus Selector1/2 -> "const delay "/2(konf)  "<ncd_delay>"
  Bus Selector/1 -> saturation/3(enable)  "<sat_schedule>"
  Bus Selector/2 -> "const delay "/3(enable)  "<ncd_schedule>"
  Bus Selector/3 -> "time correlated delay "/3(enable)  "<tcd_schedule>"
  Bus Creator/1 -> amplitude_port/1  "ffi_ampl_bus"
  "const delay "/2(delay) -> Bus Creator/2  "ncd_ampl"
  "time correlated delay "/2(delay) -> Bus Creator/3  "tcd_ampl"

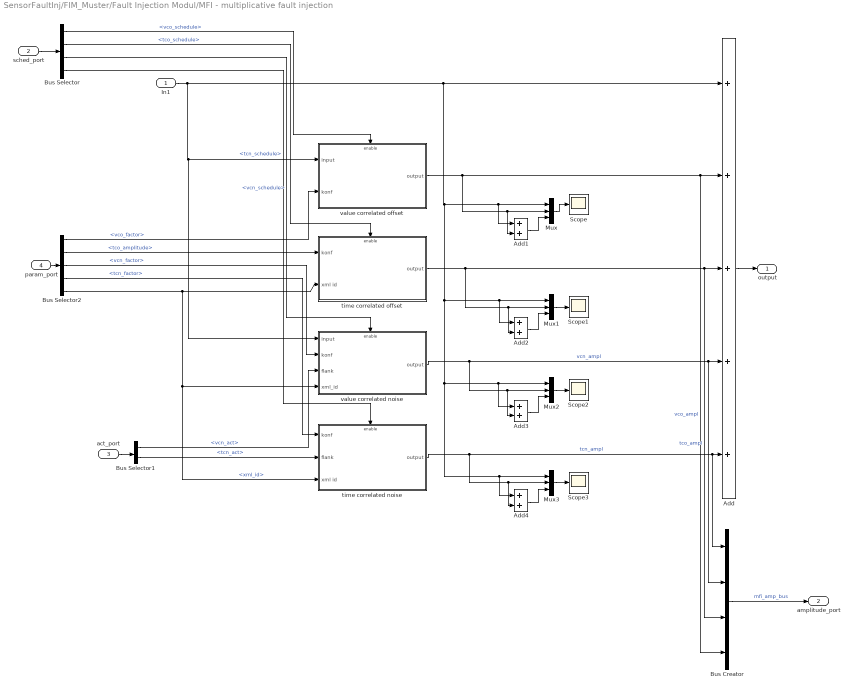
== system SensorFaultInj/FIM_Muster/Fault Injection Modul/MFI - multiplicative fault injection ==
  In1 : Inport
  sched_port : Inport  Port=2
  act_port : Inport  Port=3
  param_port : Inport  Port=4
  Add : Sum  Inputs=+++++  SampleTime=SampleTime
  Add1 : Sum
  Add2 : Sum
  Add3 : Sum  SampleTime=SampleTime
  Add4 : Sum  SampleTime=SampleTime
  Bus Creator : BusCreator
  Bus Selector : BusSelector  OutputSignals=vco_schedule,tco_schedule,vcn_schedule,tcn_schedule
  Bus Selector1 : BusSelector  OutputSignals=vcn_act,tcn_act
  Bus Selector2 : BusSelector  OutputSignals=vco_factor,tco_amplitude,vcn_factor,tcn_factor,xml_id
  Mux{,1..3} (4 alike) : Mux  Inputs=3
  Scope{,1..3} (4 alike) : Scope
      Scope settings: YMin=-55  YMax=55  SaveName=ScopeData8
      Scope1 settings: YMin=-50  YMax=55  SaveName=ScopeData11  MaxDataPoints=10000
      Scope2 settings: YMin=-70  YMax=70  SaveName=ScopeData12
      Scope3 settings: YMin=-50  YMax=60  SaveName=ScopeData13
  time correlated noise : Subsystem  TreatAsAtomicUnit=on
  time correlated offset : Subsystem  TreatAsAtomicUnit=on
  value correlated noise : Subsystem
  value correlated offset : Subsystem  TreatAsAtomicUnit=on
  output : Outport
  "amplitude_port " : Outport  Port=2
  wires:
  In1/1 -> Mux3/1, Add4/1, Mux2/1, Add3/1, Mux1/1, Add2/1, Mux/1, Add1/1, Add/1, value correlated noise/1(input), value correlated offset/1(input)
  value correlated offset/1(output) -> Bus Creator/4, Add/2, Add1/2, Mux/2  "vco_ampl"
  time correlated offset/1(output) -> Add2/2, Mux1/2, Bus Creator/3, Add/3  "tco_ampl"
  value correlated noise/1(output) -> Add3/2, Mux2/2, Bus Creator/2, Add/4  "vcn_ampl"
  time correlated noise/1(output) -> Add4/2, Mux3/2, Bus Creator/1, Add/5  "tcn_ampl"
  Mux/1 -> Scope/1
  Mux1/1 -> Scope1/1
  Mux2/1 -> Scope2/1
  Mux3/1 -> Scope3/1
  Add1/1 -> Mux/3
  Add2/1 -> Mux1/3
  Add3/1 -> Mux2/3
  Add4/1 -> Mux3/3
  Add/1 -> output/1
  sched_port/1 -> Bus Selector/1
  Bus Selector/1 -> value correlated offset/Enable  "<vco_schedule>"
  Bus Selector/2 -> time correlated offset/Enable  "<tco_schedule>"
  Bus Selector/3 -> value correlated noise/Enable  "<vcn_schedule>"
  Bus Selector/4 -> time correlated noise/Enable  "<tcn_schedule>"
  act_port/1 -> Bus Selector1/1
  Bus Selector1/2 -> time correlated noise/2(flank)  "<tcn_act>"
  Bus Selector1/1 -> value correlated noise/3(flank)  "<vcn_act>"
  param_port/1 -> Bus Selector2/1
  Bus Selector2/5 -> value correlated noise/4(xml_id), time correlated noise/3(xml id), time correlated offset/2(xml id)  "<xml_id>"
  Bus Selector2/1 -> value correlated offset/2(konf)  "<vco_factor>"
  Bus Selector2/2 -> time correlated offset/1(konf)  "<tco_amplitude>"
  Bus Selector2/3 -> value correlated noise/2(konf)  "<vcn_factor>"
  Bus Selector2/4 -> time correlated noise/1(konf)  "<tcn_factor>"
  Bus Creator/1 -> "amplitude_port "/1  "mfi_amp_bus"

== system SensorFaultInj/FIM_Muster/Fault Injection Modul/activation bus creator ==
  act_port : Inport
  Bus Selector : BusSelector  OutputSignals=vcn_act,tcn_act  OutputAsBus=on
  Bus Selector1 : BusSelector  OutputSignals=ncn_act,out_act,spi_act,stz_act,stx_act  OutputAsBus=on
  mfi_act_port : Outport
  afi_act_port : Outport  Port=2
  wires:
  act_port/1 -> Bus Selector1/1, Bus Selector/1
  Bus Selector/1 -> mfi_act_port/1  "mfi_act_bus"
  Bus Selector1/1 -> afi_act_port/1  "afi_act_bus"

== system SensorFaultInj/FIM_Muster/Fault Injection Modul/schedule bus creator ==
  schedule_port : Inport
  Bus Selector : BusSelector  OutputSignals=vco_schedule,tco_schedule,vcn_schedule,tcn_schedule  OutputAsBus=on
  Bus Selector1 : BusSelector  OutputSignals=nco_schedule,ncn_schedule,spi_schedule,out_schedule,stz_schedule,stx_schedule  OutputAsBus=on
  Bus Selector2 : BusSelector  OutputSignals=sat_schedule,ncd_schedule,tcd_schedule  OutputAsBus=on
  mfi_sched_port : Outport
  afi_sched_port : Outport  Port=2
  ffi_sched_port : Outport  Port=3
  wires:
  schedule_port/1 -> Bus Selector2/1, Bus Selector1/1, Bus Selector/1
  Bus Selector/1 -> mfi_sched_port/1  "mfi_sched_bus"
  Bus Selector1/1 -> afi_sched_port/1  "afi_sched_bus"
  Bus Selector2/1 -> ffi_sched_port/1  "ffi_sched_bus"

== system SensorFaultInj/FIM_Muster/Fault Injection Modul/schedule bus creator1 ==
  schedule_port : Inport
  Bus Selector : BusSelector  OutputSignals=parameter_bus.vco_factor,parameter_bus.tco_amplitude,parameter_bus.vcn_factor,parameter_bus.tcn_factor,xml_id  OutputAsBus=on
  Bus Selector1 : BusSelector  OutputSignals=parameter_bus.nco_amplitude,parameter_bus.ncn_factor,parameter_bus.out_param_bus,parameter_bus.spi_param_bus,parameter_bus.stx_param_bus,xml_id  OutputAsBus=on
  Bus Selector2 : BusSelector  OutputSignals=parameter_bus.sat_param_bus,parameter_bus.ncd_delay,parameter_bus.tcd_delay,xml_id  OutputAsBus=on
  mfi_sched_port : Outport
  afi_sched_port : Outport  Port=2
  ffi_sched_port : Outport  Port=3
  wires:
  schedule_port/1 -> Bus Selector2/1, Bus Selector1/1, Bus Selector/1
  Bus Selector/1 -> mfi_sched_port/1  "mfi_sched_bus"
  Bus Selector1/1 -> afi_sched_port/1  "afi_sched_bus"
  Bus Selector2/1 -> ffi_sched_port/1  "ffi_sched_bus"

== system SensorFaultInj/FIM_Muster/Local Activation Generator/Subsystem2 ==
  In1 : Inport
  In2 : Inport  Port=2
  In3 : Inport  Port=3
  0 : Logic  Operator=OR  AllPortsSameDT=off  OutDataTypeStr=boolean
  1 : Logic  Operator=OR  AllPortsSameDT=off  OutDataTypeStr=boolean
  2 : Logic  Operator=OR  AllPortsSameDT=off  OutDataTypeStr=boolean
  Switch : Switch  Threshold=1
  Switch1 : Switch  Threshold=1
  Switch2 : Switch  Threshold=1
  zero : Constant  Value=0  OutDataTypeStr=boolean
  Out1 : Outport
  Out2 : Outport  Port=2
  Out3 : Outport  Port=3
  wires:
  In1/1 -> Switch/3
  zero/1 -> Switch2/1, Switch1/1, Switch/1
  0/1 -> Switch/2
  Switch/1 -> 1/1, 2/1, Out1/1
  In3/1 -> Switch2/3
  In2/1 -> Switch1/3
  Switch1/1 -> 0/2, 2/2, Out2/1
  Switch2/1 -> 1/2, 0/1, Out3/1
  1/1 -> Switch1/2
  2/1 -> Switch2/2

== system SensorFaultInj/FIM_Muster/Local Activation Generator/bus_counter ==
  In1 : Inport
  Bus Creator : BusCreator  Inputs=7
  Bus Selector : BusSelector  OutputSignals=vcn_act,tcn_act,ncn_act,out_act,spi_act,stz_act,stx_act
  Counter{,1..3} (4 alike) : dspswit3/Counter  Direction=Up  CountEvent=Non-zero sample  CounterSize=User defined  MaxCount=10000  InitialCount=0  Output=Count  HitValue=32  ResetInput=on  SamplesPerFrame=1  Ts=1  CntDtype=double  HitDtype=Logical
  Counter4 : dspswit3/Counter  Direction=Up  CountEvent=Rising edge  CounterSize=User defined  MaxCount=10000  InitialCount=0  Output=Count  HitValue=32  ResetInput=on  SamplesPerFrame=1  Ts=1  CntDtype=double  HitDtype=Logical
  Counter5 : dspswit3/Counter  Direction=Up  CountEvent=Rising edge  CounterSize=User defined  MaxCount=10000  InitialCount=0  Output=Count  HitValue=32  ResetInput=on  SamplesPerFrame=1  Ts=1  CntDtype=double  HitDtype=Logical
  Counter6 : dspswit3/Counter  Direction=Up  CountEvent=Rising edge  CounterSize=User defined  MaxCount=10000  InitialCount=0  Output=Count  HitValue=32  ResetInput=on  SamplesPerFrame=1  Ts=1  CntDtype=double  HitDtype=Logical
  zero : Constant  Value=0  OutDataTypeStr=boolean
  Out1 : Outport
  wires:
  In1/1 -> Bus Selector/1
  Bus Selector/1 -> Counter/1  "<vcn_act>"
  Counter/1 -> Bus Creator/1
  Counter1/1 -> Bus Creator/2
  Bus Selector/2 -> Counter1/1  "<tcn_act>"
  Bus Selector/3 -> Counter2/1  "<ncn_act>"
  Bus Selector/4 -> Counter3/1  "<out_act>"
  Bus Selector/5 -> Counter4/1  "<spi_act>"
  Bus Selector/6 -> Counter5/1  "<stz_act>"
  Bus Selector/7 -> Counter6/1  "<stx_act>"
  Counter3/1 -> Bus Creator/4
  Counter4/1 -> Bus Creator/5
  Counter6/1 -> Bus Creator/7
  Counter5/1 -> Bus Creator/6
  Counter2/1 -> Bus Creator/3
  Bus Creator/1 -> Out1/1
  zero/1 -> Counter1/2, Counter6/2, Counter5/2, Counter4/2, Counter3/2, Counter2/2, Counter/2

== system SensorFaultInj/FIM_Muster/Local Activation Generator/disable non active trigger ==
  vec_probability : Inport
  vec_activation : Inport  Port=2
  Bus Creator : BusCreator  Inputs=7
  Bus Selector : BusSelector  OutputSignals=vcn_occ,tcn_occ,ncn_occ,out_occ,spi_occ,stz_occ,stx_occ
  Bus Selector1 : BusSelector  OutputSignals=vcn_schedule,tcn_schedule,ncn_schedule,out_schedule,spi_schedule,stz_schedule,stx_schedule
  Constant : Constant  Value=0
  Switch{,1..6} (7 alike) : Switch  Threshold=1
  vec_probability_ad : Outport
  wires:
  vec_probability/1 -> Bus Selector/1
  vec_activation/1 -> Bus Selector1/1
  Bus Selector1/1 -> Switch/2  "<vcn_schedule>"
  Bus Selector1/2 -> Switch1/2  "<tcn_schedule>"
  Bus Selector1/3 -> Switch2/2  "<ncn_schedule>"
  Bus Selector1/4 -> Switch3/2  "<out_schedule>"
  Bus Selector1/5 -> Switch6/2  "<spi_schedule>"
  Bus Selector1/6 -> Switch5/2  "<stz_schedule>"
  Bus Selector1/7 -> Switch4/2  "<stx_schedule>"
  Bus Selector/1 -> Switch/1  "<vcn_occ>"
  Bus Selector/2 -> Switch1/1  "<tcn_occ>"
  Bus Selector/3 -> Switch2/1  "<ncn_occ>"
  Bus Selector/4 -> Switch3/1  "<out_occ>"
  Bus Selector/5 -> Switch6/1  "<spi_occ>"
  Constant/1 -> Switch4/3, Switch5/3, Switch6/3, Switch3/3, Switch2/3, Switch1/3, Switch/3
  Switch/1 -> Bus Creator/1  "vcn_occ"
  Switch1/1 -> Bus Creator/2  "tcn_occ"
  Switch2/1 -> Bus Creator/3  "ncn_occ"
  Switch3/1 -> Bus Creator/4  "out_occ"
  Switch6/1 -> Bus Creator/5  "spi_occ"
  Switch5/1 -> Bus Creator/6  "stz_occ"
  Switch4/1 -> Bus Creator/7  "stx_occ"
  Bus Selector/7 -> Switch4/1  "<stx_occ>"
  Bus Selector/6 -> Switch5/1  "<stz_occ>"
  Bus Creator/1 -> vec_probability_ad/1

== system SensorFaultInj/FIM_Muster/Local Activation Generator/flank to dlock0 ==
  flank : Inport
  delay : Inport  Port=2
  Constant : Constant
  Constant1 : Constant  Value=0
  Counter2 : dspswit3/Counter  Direction=Up  CountEvent=Rising edge  CounterSize=User defined  MaxCount=512  InitialCount=0  Output=Count and Hit  HitValue=1  ResetInput=on  SamplesPerFrame=1  Ts=-1  CntDtype=double  HitDtype=Boolean
  Switch : Switch  Criteria=u2 > Threshold
  Unit Delay : UnitDelay  SampleTime=-1
  Variable Time Delay : VariableTransportDelay  MaximumDelay=512  ZeroDelay=on
  conv0 : DataTypeConversion  OutDataTypeStr=boolean
  conv1 : DataTypeConversion  OutDataTypeStr=double
  flag1 : Switch  Threshold=1
  block : Outport
  wires:
  Constant/1 -> flag1/1, Switch/1
  Constant1/1 -> Switch/3, flag1/3
  flank/1 -> Switch/2
  Switch/1 -> Counter2/1
  Counter2/1 -> flag1/2
  delay/1 -> Variable Time Delay/2
  Variable Time Delay/1 -> Unit Delay/1
  flag1/1 -> block/1
  conv0/1 -> Counter2/2
  Counter2/2 -> conv1/1
  conv1/1 -> Variable Time Delay/1
  Unit Delay/1 -> conv0/1

== system SensorFaultInj/FIM_Muster/Local Activation Generator/flank to dlock1 ==
  flank : Inport
  delay : Inport  Port=2
  Constant : Constant
  Constant1 : Constant  Value=0
  Counter2 : dspswit3/Counter  Direction=Up  CountEvent=Rising edge  CounterSize=User defined  MaxCount=512  InitialCount=0  Output=Count and Hit  HitValue=1  ResetInput=on  SamplesPerFrame=1  Ts=-1  CntDtype=double  HitDtype=Boolean
  Switch : Switch  Criteria=u2 > Threshold
  Unit Delay : UnitDelay  SampleTime=-1
  Variable Time Delay : VariableTransportDelay  MaximumDelay=512  ZeroDelay=on
  conv0 : DataTypeConversion  OutDataTypeStr=boolean
  conv1 : DataTypeConversion  OutDataTypeStr=double
  flag1 : Switch  Threshold=1
  block : Outport
  wires:
  Constant/1 -> flag1/1, Switch/1
  Constant1/1 -> Switch/3, flag1/3
  flank/1 -> Switch/2
  Switch/1 -> Counter2/1
  Counter2/1 -> flag1/2
  delay/1 -> Variable Time Delay/2
  Variable Time Delay/1 -> Unit Delay/1
  flag1/1 -> block/1
  conv0/1 -> Counter2/2
  Counter2/2 -> conv1/1
  conv1/1 -> Variable Time Delay/1
  Unit Delay/1 -> conv0/1

== system SensorFaultInj/FIM_Muster/Local Activation Generator/flank to dlock2 ==
  flank : Inport
  delay : Inport  Port=2
  Constant : Constant
  Constant1 : Constant  Value=0
  Counter2 : dspswit3/Counter  Direction=Up  CountEvent=Rising edge  CounterSize=User defined  MaxCount=512  InitialCount=0  Output=Count and Hit  HitValue=1  ResetInput=on  SamplesPerFrame=1  Ts=-1  CntDtype=double  HitDtype=Boolean
  Switch : Switch  Criteria=u2 > Threshold
  Unit Delay : UnitDelay  SampleTime=-1
  Variable Time Delay : VariableTransportDelay  MaximumDelay=512  ZeroDelay=on
  conv0 : DataTypeConversion  OutDataTypeStr=boolean
  conv1 : DataTypeConversion  OutDataTypeStr=double
  flag1 : Switch  Threshold=1
  block : Outport
  wires:
  Constant/1 -> flag1/1, Switch/1
  Constant1/1 -> Switch/3, flag1/3
  flank/1 -> Switch/2
  Switch/1 -> Counter2/1
  Counter2/1 -> flag1/2
  delay/1 -> Variable Time Delay/2
  Variable Time Delay/1 -> Unit Delay/1
  flag1/1 -> block/1
  conv0/1 -> Counter2/2
  Counter2/2 -> conv1/1
  conv1/1 -> Variable Time Delay/1
  Unit Delay/1 -> conv0/1

== system SensorFaultInj/FIM_Muster/Parser Modul/Fault Parameter Parser ==
  In1 : Inport
  Add1 : Sum
  Constant1 : Constant
  Digital Clock2 : DigitalClock  SampleTime=SampleTime
  Enabled Subsystem : Subsystem  TreatAsAtomicUnit=on
  Memory2 : Memory
  Subtract2 : Sum  Inputs=+-
  Out1 : Outport
  wires:
  Digital Clock2/1 -> Add1/2
  Memory2/1 -> Subtract2/2
  Constant1/1 -> Add1/1, Subtract2/1
  Add1/1 -> Memory2/1
  Subtract2/1 -> Enabled Subsystem/Enable
  In1/1 -> Enabled Subsystem/1(In1)
  Enabled Subsystem/1(Out1) -> Out1/1

== system SensorFaultInj/FIM_Muster/Parser Modul/Occurence Parser  ==
  In1 : Inport
  Add1 : Sum
  Constant1 : Constant
  Digital Clock2 : DigitalClock  SampleTime=SampleTime
  Enabled Subsystem : Subsystem  TreatAsAtomicUnit=on
  Memory2 : Memory
  Subtract2 : Sum  Inputs=+-
  Out1 : Outport
  wires:
  Digital Clock2/1 -> Add1/2
  Memory2/1 -> Subtract2/2
  Constant1/1 -> Add1/1, Subtract2/1
  Add1/1 -> Memory2/1
  Subtract2/1 -> Enabled Subsystem/Enable
  Enabled Subsystem/1(Out1) -> Out1/1
  In1/1 -> Enabled Subsystem/1(In1)

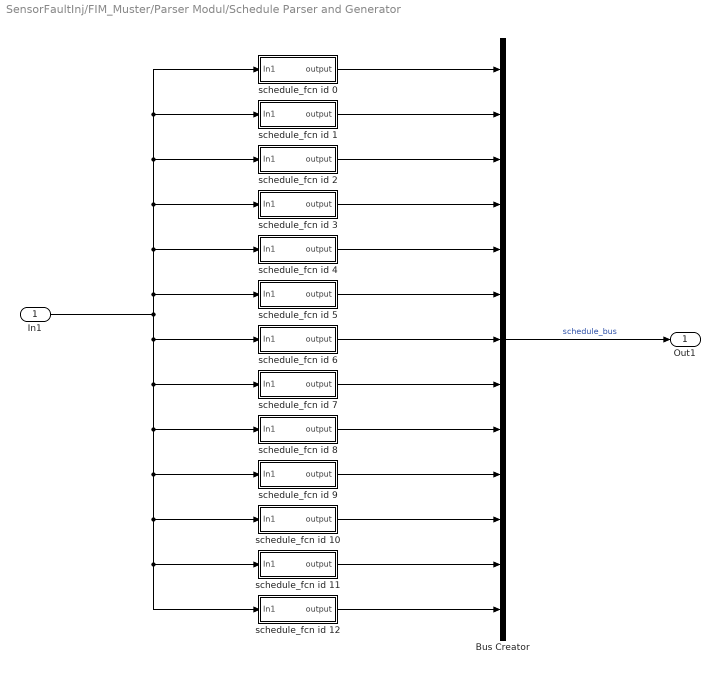
== system SensorFaultInj/FIM_Muster/Parser Modul/Schedule Parser and Generator  ==
  In1 : Inport
  Bus Creator : BusCreator  Inputs=13
  schedule_fcn id 0 : Subsystem
  schedule_fcn id 1 : Subsystem
  schedule_fcn id 10 : Subsystem
  schedule_fcn id 11 : Subsystem
  schedule_fcn id 12 : Subsystem
  schedule_fcn id 2 : Subsystem
  schedule_fcn id 3 : Subsystem
  schedule_fcn id 4 : Subsystem
  schedule_fcn id 5 : Subsystem
  schedule_fcn id 6 : Subsystem
  schedule_fcn id 7 : Subsystem
  schedule_fcn id 8 : Subsystem
  schedule_fcn id 9 : Subsystem
  Out1 : Outport
  wires:
  schedule_fcn id 3/1(output) -> Bus Creator/4
  schedule_fcn id 6/1(output) -> Bus Creator/7
  schedule_fcn id 4/1(output) -> Bus Creator/5
  schedule_fcn id 1/1(output) -> Bus Creator/2
  schedule_fcn id 0/1(output) -> Bus Creator/1
  schedule_fcn id 10/1(output) -> Bus Creator/11
  schedule_fcn id 5/1(output) -> Bus Creator/6
  schedule_fcn id 9/1(output) -> Bus Creator/10
  schedule_fcn id 8/1(output) -> Bus Creator/9
  schedule_fcn id 7/1(output) -> Bus Creator/8
  schedule_fcn id 12/1(output) -> Bus Creator/13
  schedule_fcn id 11/1(output) -> Bus Creator/12
  schedule_fcn id 2/1(output) -> Bus Creator/3
  Bus Creator/1 -> Out1/1  "schedule_bus"
  In1/1 -> schedule_fcn id 5/1(In1), schedule_fcn id 4/1(In1), schedule_fcn id 3/1(In1), schedule_fcn id 2/1(In1), schedule_fcn id 1/1(In1), schedule_fcn id 0/1(In1), schedule_fcn id 6/1(In1), schedule_fcn id 7/1(In1), schedule_fcn id 8/1(In1), schedule_fcn id 9/1(In1), schedule_fcn id 10/1(In1), schedule_fcn id 12/1(In1), schedule_fcn id 11/1(In1)

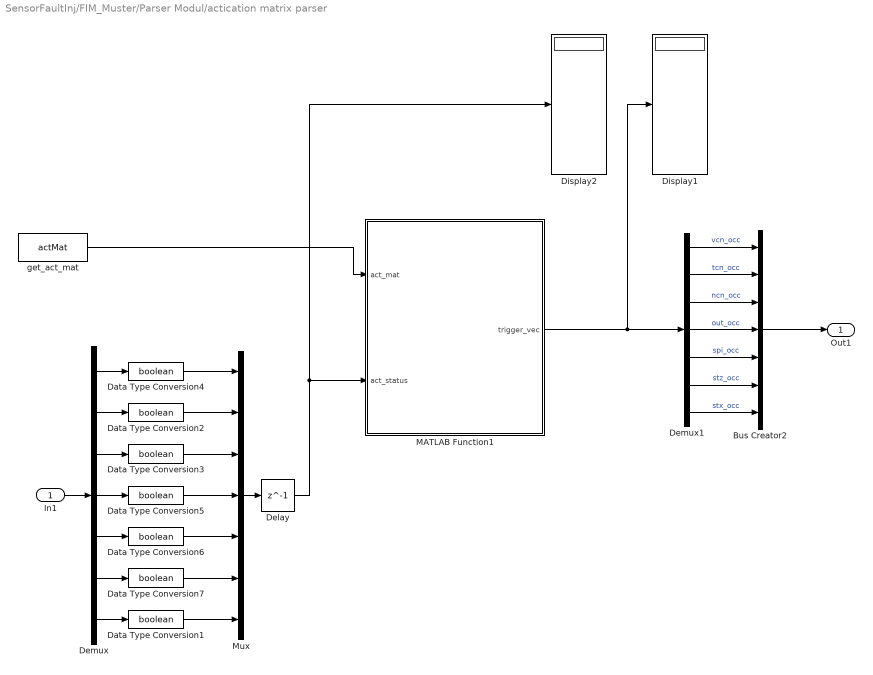
== system SensorFaultInj/FIM_Muster/Parser Modul/actication matrix parser  ==
  In1 : Inport
  Bus Creator2 : BusCreator  Inputs=7
  Data Type Conversion{1..7} (7 alike) : DataTypeConversion  OutDataTypeStr=boolean
  Delay : Delay  DelayLength=1  InitialCondition=0
  Demux : Demux  Outputs=7
  Demux1 : Demux  Outputs=7
  Display1 : Display
  Display2 : Display
  MATLAB Function1 : MATLAB Function  TreatAsAtomicUnit=on
  Mux : Mux  Inputs=7
  "get_act_mat " : Constant  Value=actMat
  Out1 : Outport  LockScale=on
  wires:
  In1/1 -> Demux/1
  "get_act_mat "/1 -> MATLAB Function1/1(act_mat)
  Data Type Conversion4/1 -> Mux/1
  Demux/1 -> Data Type Conversion4/1
  Demux/7 -> Data Type Conversion1/1
  Data Type Conversion1/1 -> Mux/7
  Demux/2 -> Data Type Conversion2/1
  Data Type Conversion2/1 -> Mux/2
  Demux/3 -> Data Type Conversion3/1
  Data Type Conversion3/1 -> Mux/3
  Demux/4 -> Data Type Conversion5/1
  Data Type Conversion5/1 -> Mux/4
  Demux/5 -> Data Type Conversion6/1
  Data Type Conversion6/1 -> Mux/5
  Demux/6 -> Data Type Conversion7/1
  Data Type Conversion7/1 -> Mux/6
  Mux/1 -> Delay/1
  MATLAB Function1/1(trigger_vec) -> Demux1/1, Display1/1
  Demux1/1 -> Bus Creator2/1  "vcn_occ"
  Demux1/2 -> Bus Creator2/2  "tcn_occ"
  Demux1/3 -> Bus Creator2/3  "ncn_occ"
  Demux1/4 -> Bus Creator2/4  "out_occ"
  Demux1/5 -> Bus Creator2/5  "spi_occ"
  Demux1/6 -> Bus Creator2/6  "stz_occ"
  Demux1/7 -> Bus Creator2/7  "stx_occ"
  Bus Creator2/1 -> Out1/1
  Delay/1 -> Display2/1, MATLAB Function1/2(act_status)

== system SensorFaultInj/Glogal Activation Generator/Enabled Subsystem/global parser2 ==
  ex_sfun_globalocc : S-Function  FunctionName=ex_sfun_globalocc  EnableBusSupport=off  mask(Legacy Function){SFunctionSpec=double y1 = global_occ(single u1), ShowSpec=on}
      mask prompts: ShowSpec "Display function specification"
      mask help:
      | This block allows you to call the legacy functions specified by the following Legacy Code Tool definition:
      | def.SFunctionName = 'ex_sfun_globalocc';
      | def.OutputFcnSpec = 'double y1 = global_occ(single u1)';
      | def.HeaderFiles = {'global_occ.hpp'};
      | def.SourceFiles = {'global_occ.cpp'};
      | def.Options.language = 'C++';
      mask Help: <p>This block was generated automatically by the Legacy Code Tool. For detailed help on this tool, call<a href="matlab:legacy_code('help')"> legacy_code('help')</a>.</p>
      mask Callback ShowSpec:
      | if strcmp(get_param(gcbh, 'ShowSpec'), 'on')
      |   set_param(gcbh, 'MaskDisplay', sprintf('fprintf(''%s'');', get_param(gcbh, 'SFunctionSpec')));
      | else
      |   set_param(gcbh, 'MaskDisplay', sprintf('fprintf(''%s'');', get_param(gcbh, 'FunctionName')));
      | end
      mask Display: fprintf('double y1 = global_occ(single u1)');
  fault id : Constant  Value=2  OutDataTypeStr=single
  occ : Outport
  wires:
  ex_sfun_globalocc/1 -> occ/1  "glo_vcn_occ"
  fault id/1 -> ex_sfun_globalocc/1

== system SensorFaultInj/Glogal Activation Generator/Enabled Subsystem/global parser3 ==
  ex_sfun_globalocc : S-Function  FunctionName=ex_sfun_globalocc  EnableBusSupport=off  mask(Legacy Function){SFunctionSpec=double y1 = global_occ(single u1), ShowSpec=on}
      mask prompts: ShowSpec "Display function specification"
      mask help:
      | This block allows you to call the legacy functions specified by the following Legacy Code Tool definition:
      | def.SFunctionName = 'ex_sfun_globalocc';
      | def.OutputFcnSpec = 'double y1 = global_occ(single u1)';
      | def.HeaderFiles = {'global_occ.hpp'};
      | def.SourceFiles = {'global_occ.cpp'};
      | def.Options.language = 'C++';
      mask Help: <p>This block was generated automatically by the Legacy Code Tool. For detailed help on this tool, call<a href="matlab:legacy_code('help')"> legacy_code('help')</a>.</p>
      mask Callback ShowSpec:
      | if strcmp(get_param(gcbh, 'ShowSpec'), 'on')
      |   set_param(gcbh, 'MaskDisplay', sprintf('fprintf(''%s'');', get_param(gcbh, 'SFunctionSpec')));
      | else
      |   set_param(gcbh, 'MaskDisplay', sprintf('fprintf(''%s'');', get_param(gcbh, 'FunctionName')));
      | end
      mask Display: fprintf('double y1 = global_occ(single u1)');
  fault id : Constant  Value=3  OutDataTypeStr=single
  occ : Outport
  wires:
  ex_sfun_globalocc/1 -> occ/1  "glo_tcn_occ"
  fault id/1 -> ex_sfun_globalocc/1

== system SensorFaultInj/Glogal Activation Generator/Enabled Subsystem/global parser5 ==
  ex_sfun_globalocc : S-Function  FunctionName=ex_sfun_globalocc  EnableBusSupport=off  mask(Legacy Function){SFunctionSpec=double y1 = global_occ(single u1), ShowSpec=on}
      mask prompts: ShowSpec "Display function specification"
      mask help:
      | This block allows you to call the legacy functions specified by the following Legacy Code Tool definition:
      | def.SFunctionName = 'ex_sfun_globalocc';
      | def.OutputFcnSpec = 'double y1 = global_occ(single u1)';
      | def.HeaderFiles = {'global_occ.hpp'};
      | def.SourceFiles = {'global_occ.cpp'};
      | def.Options.language = 'C++';
      mask Help: <p>This block was generated automatically by the Legacy Code Tool. For detailed help on this tool, call<a href="matlab:legacy_code('help')"> legacy_code('help')</a>.</p>
      mask Callback ShowSpec:
      | if strcmp(get_param(gcbh, 'ShowSpec'), 'on')
      |   set_param(gcbh, 'MaskDisplay', sprintf('fprintf(''%s'');', get_param(gcbh, 'SFunctionSpec')));
      | else
      |   set_param(gcbh, 'MaskDisplay', sprintf('fprintf(''%s'');', get_param(gcbh, 'FunctionName')));
      | end
      mask Display: fprintf('double y1 = global_occ(single u1)');
  fault id : Constant  Value=5  OutDataTypeStr=single
  occ : Outport
  wires:
  ex_sfun_globalocc/1 -> occ/1  "glo_ncn_occ"
  fault id/1 -> ex_sfun_globalocc/1
